simulink model "DT_UDE_Obs"  (R2021a)
settings: Solver=ode4  StartTime=0.0  StopTime=tstop  FixedStep=Ts  RelTol=1e-3
values from neighbouring files (symbols this model uses):
  K = place(F_n, G_n, eig(F_m))    [data.m]
  Ts = 0.001    [data.m]
  udic = (-Ts/T)*pinv(G_n)*ehatic    [data.m]
  xhatic = zeros(4, 1)    [data.m]
  xic = zeros(4, 1)    [data.m]
  xmic = zeros(4, 1)    [data.m]
undefined symbols (not defined in the file or in its folder): operric
settings Model: Creator=Ram Padmanabhan  LastModifiedBy=Ram Padmanabhan
settings SolverCC: AlgebraicLoopSolver=TrustRegion
settings DataIOCC: SaveOutput=off  SignalLogging=off  DSMLogging=off  SaveTime=off  ReturnWorkspaceOutputs=off
settings DebuggingCC: SFMachineParentedDataDiag=warning

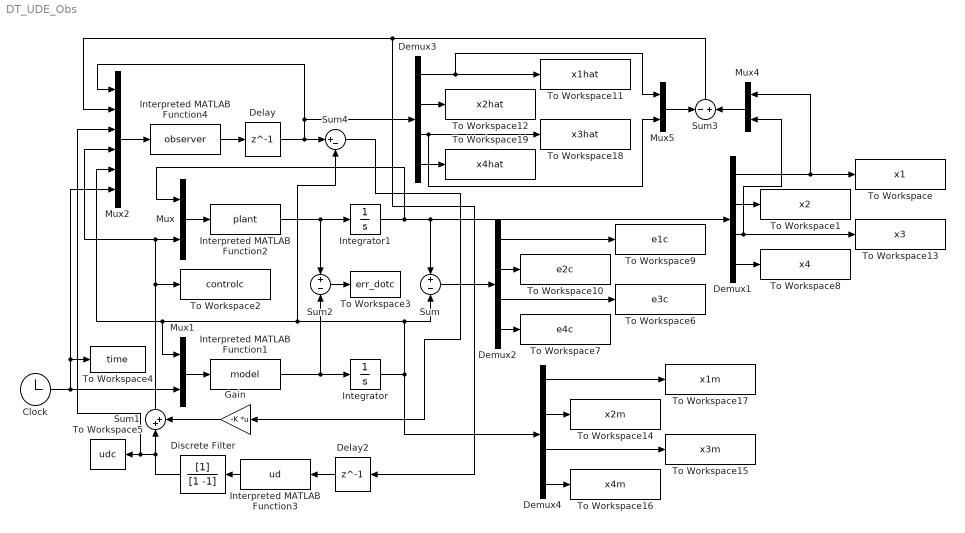
== system DT_UDE_Obs ==
  Clock : Clock
  Delay : Delay  DelayLength=1  InitialCondition=xhatic  SampleTime=Ts
  Delay2 : Delay  DelayLength=1  InitialCondition=operric  SampleTime=Ts
  Demux{1..4} (4 alike) : Demux
  Discrete Filter : DiscreteFilter  Denominator=[1 -1]  InitialStates=udic  SampleTime=Ts
  Gain : Gain  Gain=-K  Multiplication=Matrix(K*u)
  Integrator : Integrator  InitialCondition=xmic
  Integrator1 : Integrator  InitialCondition=xic
  Interpreted MATLAB Function1 : MATLABFcn  MATLABFcn=model  OutputDimensions=4
  Interpreted MATLAB Function2 : MATLABFcn  MATLABFcn=plant  OutputDimensions=4
  Interpreted MATLAB Function3 : MATLABFcn  MATLABFcn=ud  OutputDimensions=2
  Interpreted MATLAB Function4 : MATLABFcn  MATLABFcn=observer  OutputDimensions=4
  Mux{,1,4..5} (4 alike) : Mux  Inputs=2
  Mux2 : Mux  Inputs=6
  Sum : Sum  Inputs=+-
  Sum1 : Sum  Inputs=|++
  Sum2 : Sum  Inputs=+-
  Sum3 : Sum  Inputs=-+
  Sum4 : Sum  Inputs=|+-
  To Workspace : ToWorkspace  VariableName=x1  SampleTime=-1
  To Workspace1 : ToWorkspace  VariableName=x2  SampleTime=-1
  To Workspace10 : ToWorkspace  VariableName=e2c  SampleTime=-1
  To Workspace11 : ToWorkspace  VariableName=x1hat  SampleTime=-1
  To Workspace12 : ToWorkspace  VariableName=x2hat  SampleTime=-1
  To Workspace13 : ToWorkspace  VariableName=x3  SampleTime=-1
  To Workspace14 : ToWorkspace  VariableName=x2m  SampleTime=-1
  To Workspace15 : ToWorkspace  VariableName=x3m  SampleTime=-1
  To Workspace16 : ToWorkspace  VariableName=x4m  SampleTime=-1
  To Workspace17 : ToWorkspace  VariableName=x1m  SampleTime=-1
  To Workspace18 : ToWorkspace  VariableName=x3hat  SampleTime=-1
  To Workspace19 : ToWorkspace  VariableName=x4hat  SampleTime=-1
  To Workspace2 : ToWorkspace  VariableName=controlc  SampleTime=-1
  To Workspace3 : ToWorkspace  VariableName=err_dotc  SampleTime=-1
  To Workspace4 : ToWorkspace  VariableName=time  SampleTime=-1
  To Workspace5 : ToWorkspace  VariableName=udc  SampleTime=-1
  To Workspace6 : ToWorkspace  VariableName=e3c  SampleTime=-1
  To Workspace7 : ToWorkspace  VariableName=e4c  SampleTime=-1
  To Workspace8 : ToWorkspace  VariableName=x4  SampleTime=-1
  To Workspace9 : ToWorkspace  VariableName=e1c  SampleTime=-1
  wires:
  Interpreted MATLAB Function1/1 -> Integrator/1, Sum2/2
  Mux/1 -> Interpreted MATLAB Function2/1
  Integrator1/1 -> Mux/1, Demux1/1, Sum/1
  Integrator/1 -> Demux4/1, Mux2/5, Mux1/1, Sum4/2, Sum/2
  Mux1/1 -> Interpreted MATLAB Function1/1
  Clock/1 -> Mux1/2, To Workspace4/1, Mux2/6
  Interpreted MATLAB Function2/1 -> Integrator1/1, Sum2/1
  Sum1/1 -> Mux2/4, Mux/2, To Workspace2/1
  Gain/1 -> Sum1/2
  Interpreted MATLAB Function3/1 -> Discrete Filter/1
  Delay2/1 -> Interpreted MATLAB Function3/1
  Demux1/1 -> Mux4/1, To Workspace/1
  Demux1/2 -> To Workspace1/1
  Demux2/1 -> To Workspace9/1
  Sum/1 -> Demux2/1
  Demux2/2 -> To Workspace10/1
  Discrete Filter/1 -> Mux2/3, To Workspace5/1, Sum1/1
  Sum2/1 -> To Workspace3/1
  Demux2/4 -> To Workspace7/1
  Demux2/3 -> To Workspace6/1
  Demux1/3 -> To Workspace13/1, Mux4/2
  Demux1/4 -> To Workspace8/1
  Demux4/4 -> To Workspace16/1
  Demux4/2 -> To Workspace14/1
  Demux4/1 -> To Workspace17/1
  Demux4/3 -> To Workspace15/1
  Interpreted MATLAB Function4/1 -> Delay/1
  Mux2/1 -> Interpreted MATLAB Function4/1
  Delay/1 -> Sum4/1, Demux3/1, Mux2/1
  Sum4/1 -> Gain/1
  Demux3/4 -> To Workspace19/1
  Demux3/2 -> To Workspace12/1
  Demux3/1 -> To Workspace11/1, Mux5/1
  Demux3/3 -> To Workspace18/1, Mux5/2
  Mux5/1 -> Sum3/1
  Mux4/1 -> Sum3/2
  Sum3/1 -> Delay2/1, Mux2/2
